simulink library "lib_fuel_converter3"  (Simulink 10.1)
settings: Solver=VariableStepAuto  StartTime=0.0  StopTime=10.0  RelTol=1e-3
undefined symbols (not defined in the file or in its folder): air_cp, amb_tmp, cyc_mph, ex_gas_cp, fc_acc_mass, fc_base_mass, fc_c2i_th_cond, fc_c_init_tmp, fc_cl2h_eff, fc_CO2_to_FUELgps, fc_cold, fc_cold_tmp, fc_cp, fc_ct_trq, fc_emisv, fc_ext_sarea, fc_fuel_den, fc_fuel_lhv, fc_h2x_th_cond, fc_h_air_flow, fc_h_cp, fc_h_init_tmp, fc_hood_emisv, fc_hood_sarea, fc_i2x_th_cond, fc_i_init_tmp, fc_inertia, fc_map_spd, fc_map_trq, fc_max_trq, fc_pwr_scale, fc_spd_scale, fc_trq_scale, fc_tstat, fc_x_init_tmp, fd_ratio, gb_num_init, gb_ratio, pow, vc_idle_bool, vc_idle_spd, vc_key_on, veh_glider_mass, wh_radius
undefined symbols (not defined in the file): fc_co_map, fc_co_map_c2h, fc_exflow_map, fc_extmp_map, fc_fuel_map, fc_fuel_map_c2h, fc_hc_map, fc_hc_map_c2h, fc_nn_model_name, fc_nox_map, fc_nox_map_c2h, fc_o2_map, fc_pm_map, fc_pm_map_c2h, generalName, logFlag
libraries: $bdroot x4, lib_etc x4, lib_fuel_converter x2, lib_fuel_converter2 x1
(part 4 of 8)

== system lib_fuel_converter3/configurable subsystems/fuel use and EO emis/fc temp correct/fc temp correct Variable Correction Factors (Map Based) ==
  Coolant T (C) : Inport
  HOT fuel use (g/s) : Inport  Port=2
  HOT emis (g/s) : Inport  Port=3
  T (Nm) : Inport  Port=4
  w (rad/s) : Inport  Port=5
  Enable : EnablePort  StatesWhenEnabling=reset
  (Thot-Temp) -------------------- (Thot-Tcold) : Fcn  Expr=(fc_tstat-u)/(fc_tstat-fc_cold_tmp)
  CO factor cold-to-hot : Subsystem  mask(2-D Table Lookup){xindex=fc_map_spd*fc_spd_scale, yindex=fc_map_trq*fc_trq_scale, table=fc_co_map_c2h}
      mask prompts: xindex "X Index"; yindex "Y Index"
      mask help:
      | Two Dimensional Table Lookup
      | The first input corresponds to X Index and the second input corresponds to the Y Index
      mask init:
      | sftab2chk(xindex,yindex,table);
      mask Help: This block returns a linearly interpolated intersection from the table using the X index (which corresponds to the rows of the table) and the Y index (which corresponds to the columns of the table).  Extrapolation is used.
      mask Display: plot(-10,-10,110,110,[90,50,10],[90,40,30],[90,50,10],[50,26,20],[90,50,10],[22,13,10])
  HC factor cold-to-hot : Subsystem  mask(2-D Table Lookup){xindex=fc_map_spd*fc_spd_scale, yindex=fc_map_trq*fc_trq_scale, table=fc_hc_map_c2h}
      mask prompts: xindex "X Index"; yindex "Y Index"
      mask help:
      | Two Dimensional Table Lookup
      | The first input corresponds to X Index and the second input corresponds to the Y Index
      mask init:
      | sftab2chk(xindex,yindex,table);
      mask Help: This block returns a linearly interpolated intersection from the table using the X index (which corresponds to the rows of the table) and the Y index (which corresponds to the columns of the table).  Extrapolation is used.
      mask Display: plot(-10,-10,110,110,[90,50,10],[90,40,30],[90,50,10],[50,26,20],[90,50,10],[22,13,10])
  Mux{1..5} (5 alike) : Mux  Inputs=2
  Mux6 : Mux
  NOx factor cold-to-hot : Subsystem  mask(2-D Table Lookup){xindex=fc_map_spd*fc_spd_scale, yindex=fc_map_trq*fc_trq_scale, table=fc_nox_map_c2h}
      mask prompts: xindex "X Index"; yindex "Y Index"
      mask help:
      | Two Dimensional Table Lookup
      | The first input corresponds to X Index and the second input corresponds to the Y Index
      mask init:
      | sftab2chk(xindex,yindex,table);
      mask Help: This block returns a linearly interpolated intersection from the table using the X index (which corresponds to the rows of the table) and the Y index (which corresponds to the columns of the table).  Extrapolation is used.
      mask Display: plot(-10,-10,110,110,[90,50,10],[90,40,30],[90,50,10],[50,26,20],[90,50,10],[22,13,10])
  PM factor cold-to-hot : Subsystem  mask(2-D Table Lookup){xindex=fc_map_spd*fc_spd_scale, yindex=fc_map_trq*fc_trq_scale, table=fc_pm_map_c2h}
      mask prompts: xindex "X Index"; yindex "Y Index"
      mask help:
      | Two Dimensional Table Lookup
      | The first input corresponds to X Index and the second input corresponds to the Y Index
      mask init:
      | sftab2chk(xindex,yindex,table);
      mask Help: This block returns a linearly interpolated intersection from the table using the X index (which corresponds to the rows of the table) and the Y index (which corresponds to the columns of the table).  Extrapolation is used.
      mask Display: plot(-10,-10,110,110,[90,50,10],[90,40,30],[90,50,10],[50,26,20],[90,50,10],[22,13,10])
  Product : Product  SaturateOnIntegerOverflow=on
  Product1 : Product  SaturateOnIntegerOverflow=on
  Saturation1 : Saturate  UpperLimit=max(fc_map_trq*fc_trq_scale)  LowerLimit=min(fc_map_trq*fc_trq_scale)
  Saturation2 : Saturate  UpperLimit=max(fc_map_spd*fc_spd_scale)  LowerLimit=min(fc_map_spd*fc_spd_scale)
  cold/hot =1+(factor-1) *Temp_ratio{,1..4} (5 alike) : Fcn  Expr=1+(u[2]-1)*u[1]
  fuel factor cold-to-hot : Subsystem  mask(2-D Table Lookup){xindex=fc_map_spd*fc_spd_scale, yindex=fc_map_trq*fc_trq_scale, table=fc_fuel_map_c2h}
      mask prompts: xindex "X Index"; yindex "Y Index"
      mask help:
      | Two Dimensional Table Lookup
      | The first input corresponds to X Index and the second input corresponds to the Y Index
      mask init:
      | sftab2chk(xindex,yindex,table);
      mask Help: This block returns a linearly interpolated intersection from the table using the X index (which corresponds to the rows of the table) and the Y index (which corresponds to the columns of the table).  Extrapolation is used.
      mask Display: plot(-10,-10,110,110,[90,50,10],[90,40,30],[90,50,10],[50,26,20],[90,50,10],[22,13,10])
  limit to data limits : Saturate  UpperLimit=1  LowerLimit=0
  fuel use (g/s) : Outport  OutputWhenDisabled=reset  InitialOutput=0
  EO emis (g/s) : Outport  Port=2  OutputWhenDisabled=reset  InitialOutput=0
  wires:
  cold/hot =1+(factor-1) *Temp_ratio4/1 -> Mux6/4
  cold/hot =1+(factor-1) *Temp_ratio3/1 -> Mux6/3
  cold/hot =1+(factor-1) *Temp_ratio2/1 -> Mux6/2
  cold/hot =1+(factor-1) *Temp_ratio1/1 -> Mux6/1
  cold/hot =1+(factor-1) *Temp_ratio/1 -> Product1/2
  limit to data limits/1 -> Mux5/1, Mux4/1, Mux3/1, Mux2/1, Mux1/1
  (Thot-Temp) -------------------- (Thot-Tcold)/1 -> limit to data limits/1
  Mux6/1 -> Product/1
  w (rad/s)/1 -> Saturation2/1
  T (Nm)/1 -> Saturation1/1
  HOT emis (g/s)/1 -> Product/2
  Product/1 -> EO emis (g/s)/1
  Product1/1 -> fuel use (g/s)/1
  Mux5/1 -> cold/hot =1+(factor-1) *Temp_ratio4/1
  Mux4/1 -> cold/hot =1+(factor-1) *Temp_ratio3/1
  Mux3/1 -> cold/hot =1+(factor-1) *Temp_ratio2/1
  Mux2/1 -> cold/hot =1+(factor-1) *Temp_ratio1/1
  PM factor cold-to-hot/1(table out) -> Mux5/2
  NOx factor cold-to-hot/1(table out) -> Mux4/2
  CO factor cold-to-hot/1(table out) -> Mux3/2
  HC factor cold-to-hot/1(table out) -> Mux2/2
  Mux1/1 -> cold/hot =1+(factor-1) *Temp_ratio/1
  fuel factor cold-to-hot/1(table out) -> Mux1/2
  Coolant T (C)/1 -> (Thot-Temp) -------------------- (Thot-Tcold)/1
  Saturation1/1 -> PM factor cold-to-hot/2(y0), NOx factor cold-to-hot/2(y0), CO factor cold-to-hot/2(y0), HC factor cold-to-hot/2(y0), fuel factor cold-to-hot/2(y0)
  Saturation2/1 -> PM factor cold-to-hot/1(x0), NOx factor cold-to-hot/1(x0), CO factor cold-to-hot/1(x0), HC factor cold-to-hot/1(x0), fuel factor cold-to-hot/1(x0)
  HOT fuel use (g/s)/1 -> Product1/1

== system lib_fuel_converter3/configurable subsystems/fuel use and EO emis Neural Network Model/HOT engine maps/Block NOTES ==
  note: This block determines the fully hot fuel use, engine-out emissions output rates, exhaust gas mass flow rate,
      | and engine-out exhaust gas temperature as a function of engine output torque and speed.
      | The engine maps (except for exhaust gas temperature) can be scaled using variables fc_spd_scale and
      |  fc_trq_scale; it is recommended that scaling values outside the range of 0.85 to 1.15 be used CAREFULLY.

== system lib_fuel_converter3/configurable subsystems/fuel use and EO emis Neural Network Model/HOT engine maps/CO (g/s) ==
  x0 : Inport
  y0 : Inport  Port=2
  Mux : Mux  Inputs=2
  S-function : S-Function  FunctionName=sftable2  Parameters=xindex, yindex, table  SFunctionDeploymentMode=off  EnableBusSupport=off
  table out : Outport  InitialOutput=0
  wires:
  y0/1 -> Mux/2
  S-function/1 -> table out/1
  x0/1 -> Mux/1
  Mux/1 -> S-function/1

== system lib_fuel_converter3/configurable subsystems/fuel use and EO emis Neural Network Model/HOT engine maps/HC (g/s) ==
  x0 : Inport
  y0 : Inport  Port=2
  Mux : Mux  Inputs=2
  S-function : S-Function  FunctionName=sftable2  Parameters=xindex, yindex, table  SFunctionDeploymentMode=off  EnableBusSupport=off
  table out : Outport  InitialOutput=0
  wires:
  y0/1 -> Mux/2
  S-function/1 -> table out/1
  x0/1 -> Mux/1
  Mux/1 -> S-function/1

== system lib_fuel_converter3/configurable subsystems/fuel use and EO emis Neural Network Model/HOT engine maps/MF,ex (g/s) ==
  x0 : Inport
  y0 : Inport  Port=2
  Mux : Mux  Inputs=2
  S-function : S-Function  FunctionName=sftable2  Parameters=xindex, yindex, table  SFunctionDeploymentMode=off  EnableBusSupport=off
  table out : Outport  InitialOutput=0
  wires:
  y0/1 -> Mux/2
  S-function/1 -> table out/1
  x0/1 -> Mux/1
  Mux/1 -> S-function/1

== system lib_fuel_converter3/configurable subsystems/fuel use and EO emis Neural Network Model/HOT engine maps/NOx (g/s) ==
  x0 : Inport
  y0 : Inport  Port=2
  Mux : Mux  Inputs=2
  S-function : S-Function  FunctionName=sftable2  Parameters=xindex, yindex, table  SFunctionDeploymentMode=off  EnableBusSupport=off
  table out : Outport  InitialOutput=0
  wires:
  y0/1 -> Mux/2
  S-function/1 -> table out/1
  x0/1 -> Mux/1
  Mux/1 -> S-function/1

== system lib_fuel_converter3/configurable subsystems/fuel use and EO emis Neural Network Model/HOT engine maps/O2 (g/s) ==
  x0 : Inport
  y0 : Inport  Port=2
  Mux : Mux  Inputs=2
  S-function : S-Function  FunctionName=sftable2  Parameters=xindex, yindex, table  SFunctionDeploymentMode=off  EnableBusSupport=off
  table out : Outport  InitialOutput=0
  wires:
  Mux/1 -> S-function/1
  x0/1 -> Mux/1
  S-function/1 -> table out/1
  y0/1 -> Mux/2

== system lib_fuel_converter3/configurable subsystems/fuel use and EO emis Neural Network Model/HOT engine maps/PM (g/s) ==
  x0 : Inport
  y0 : Inport  Port=2
  Mux : Mux  Inputs=2
  S-function : S-Function  FunctionName=sftable2  Parameters=xindex, yindex, table  SFunctionDeploymentMode=off  EnableBusSupport=off
  table out : Outport  InitialOutput=0
  wires:
  y0/1 -> Mux/2
  S-function/1 -> table out/1
  x0/1 -> Mux/1
  Mux/1 -> S-function/1

== system lib_fuel_converter3/configurable subsystems/fuel use and EO emis Neural Network Model/HOT engine maps/Tex,eo (C) ==
  x0 : Inport
  y0 : Inport  Port=2
  Mux : Mux  Inputs=2
  S-function : S-Function  FunctionName=sftable2  Parameters=xindex, yindex, table  SFunctionDeploymentMode=off  EnableBusSupport=off
  table out : Outport  InitialOutput=0
  wires:
  y0/1 -> Mux/2
  S-function/1 -> table out/1
  x0/1 -> Mux/1
  Mux/1 -> S-function/1

== system lib_fuel_converter3/configurable subsystems/fuel use and EO emis Neural Network Model/HOT engine maps/fuel (g/s) ==
  x0 : Inport
  y0 : Inport  Port=2
  Mux : Mux  Inputs=2
  S-function : S-Function  FunctionName=sftable2  Parameters=xindex, yindex, table  SFunctionDeploymentMode=off  EnableBusSupport=off
  table out : Outport  InitialOutput=0
  wires:
  y0/1 -> Mux/2
  S-function/1 -> table out/1
  x0/1 -> Mux/1
  Mux/1 -> S-function/1

== system lib_fuel_converter3/configurable subsystems/fuel use and EO emis Neural Network Model/fc temp/Block NOTES ==
  note: This block models the thermal behavior internal combustion engine (ICE).
      | Emphasis is on the coolant since this temperature is used to correct engine
      | fuel use.

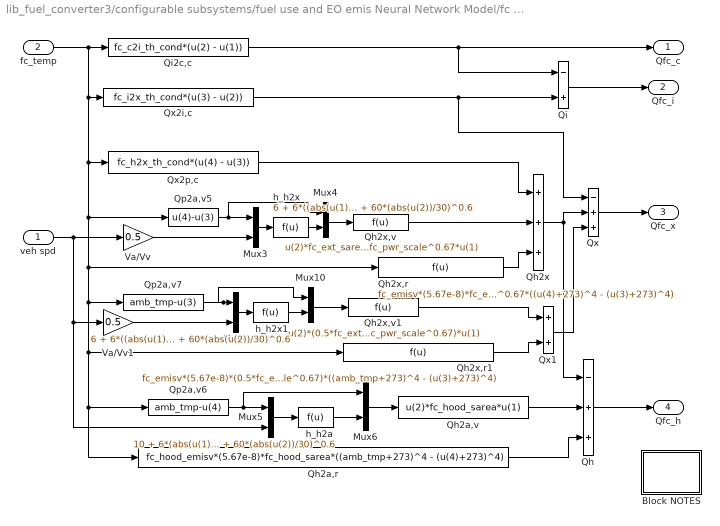
== system lib_fuel_converter3/configurable subsystems/fuel use and EO emis Neural Network Model/fc temp/fc mass heat flow ==
  veh spd : Inport
  fc_temp : Inport  Port=2
  Block NOTES : Subsystem
      mask Display: disp('Block\nNOTES')
  Mux{3..6,9..10} (6 alike) : Mux  Inputs=2
  Qh : Sum  Inputs=-++  SaturateOnIntegerOverflow=on
  Qh2a,r : Fcn  Expr=fc_hood_emisv*(5.67e-8)*fc_hood_sarea*((amb_tmp+273)^4 - (u(4)+273)^4)
  Qh2a,v : Fcn  Expr=u(2)*fc_hood_sarea*u(1)
  Qh2x : Sum  Inputs=+++  SaturateOnIntegerOverflow=on
  Qh2x,r : Fcn  Expr=fc_emisv*(5.67e-8)*fc_ext_sarea*fc_pwr_scale^0.67*((u(4)+273)^4 - (u(3)+273)^4)
  Qh2x,r1 : Fcn  Expr=fc_emisv*(5.67e-8)*(0.5*fc_ext_sarea*fc_pwr_scale^0.67)*((amb_tmp+273)^4 - (u(3)+273)^4)
  Qh2x,v : Fcn  Expr=u(2)*fc_ext_sarea*fc_pwr_scale^0.67*u(1)
  Qh2x,v1 : Fcn  Expr=u(2)*(0.5*fc_ext_sarea*fc_pwr_scale^0.67)*u(1)
  Qi : Sum  Inputs=-+  SaturateOnIntegerOverflow=on
  Qi2c,c : Fcn  Expr=fc_c2i_th_cond*(u(2) - u(1))
  Qp2a,v5 : Fcn  Expr=u(4)-u(3)
  Qp2a,v6 : Fcn  Expr=amb_tmp-u(4)
  Qp2a,v7 : Fcn  Expr=amb_tmp-u(3)
  Qx : Sum  Inputs=-++  SaturateOnIntegerOverflow=on
  Qx1 : Sum  SaturateOnIntegerOverflow=on
  Qx2i,c : Fcn  Expr=fc_i2x_th_cond*(u(3) - u(2))
  Qx2p,c : Fcn  Expr=fc_h2x_th_cond*(u(4) - u(3))
  Va/Vv : Gain  Gain=0.5  SaturateOnIntegerOverflow=on
  Va/Vv1 : Gain  Gain=0.5  SaturateOnIntegerOverflow=on
  h_h2a : Fcn  Expr=10 + 6*(abs(u(1))/1000)^0.3 + 60*(abs(u(2))/30)^0.6
  h_h2x : Fcn  Expr=6 + 6*((abs(u(1))/1000))^0.3 + 60*(abs(u(2))/30)^0.6
  h_h2x1 : Fcn  Expr=6 + 6*((abs(u(1))/1000))^0.3 + 60*(abs(u(2))/30)^0.6
  Qfc_c : Outport
  Qfc_i : Outport  Port=2
  Qfc_x : Outport  Port=3
  Qfc_h : Outport  Port=4
  wires:
  Mux10/1 -> Qh2x,v1/1
  Mux9/1 -> h_h2x1/1
  Qp2a,v7/1 -> Mux9/1, Mux10/1
  h_h2x1/1 -> Mux10/2
  Va/Vv1/1 -> Mux9/2
  Mux4/1 -> Qh2x,v/1
  Mux3/1 -> h_h2x/1
  Qp2a,v5/1 -> Mux3/1, Mux4/1
  h_h2x/1 -> Mux4/2
  veh spd/1 -> Va/Vv/1, Mux5/2, Va/Vv1/1
  Va/Vv/1 -> Mux3/2
  Qi2c,c/1 -> Qfc_c/1, Qi/1
  fc_temp/1 -> Qx2p,c/1, Qh2x,r/1, Qp2a,v7/1, Qp2a,v6/1, Qh2a,r/1, Qh2x,r1/1, Qp2a,v5/1, Qx2i,c/1, Qi2c,c/1
  Qx2i,c/1 -> Qi/2, Qx/1
  Qi/1 -> Qfc_i/1
  Qx/1 -> Qfc_x/1
  Qh2x/1 -> Qx/2, Qh/1
  Qh/1 -> Qfc_h/1
  Mux6/1 -> Qh2a,v/1
  Mux5/1 -> h_h2a/1
  Qp2a,v6/1 -> Mux5/1, Mux6/1
  h_h2a/1 -> Mux6/2
  Qx1/1 -> Qx/3
  Qh2x,v/1 -> Qh2x/2
  Qx2p,c/1 -> Qh2x/1
  Qh2x,r1/1 -> Qx1/2
  Qh2x,v1/1 -> Qx1/1
  Qh2a,r/1 -> Qh/3
  Qh2a,v/1 -> Qh/2
  Qh2x,r/1 -> Qh2x/3

== system lib_fuel_converter3/configurable subsystems/fuel use and EO emis Neural Network Model/fc temp/old fc coolant  temp. (C) ==
  fc on? : Inport
  veh spd : Inport  Port=2
  Block NOTES : Subsystem
      mask Display: disp('Block\nNOTES')
  Mux : Mux
  TEC : Integrator  InitialCondition=fc_i_init_tmp
  compute engine dT/dt : Fcn  Expr=1.1*u[1]*(-u[2]/218)*(95-u[4])+(1-u[1])*u[3]*(u[4]-amb_tmp)
  gamma (takes v as input) : Fcn  Expr=(-8.22e-5*u+8.09e-6*4-1.45e-4)*.45
  log(1-40/75) : Constant  Value=-0.7621
  fc coolant  temp (C) : Outport  InitialOutput=0
  wires:
  compute engine dT/dt/1 -> TEC/1
  gamma (takes v as input)/1 -> Mux/3
  log(1-40/75)/1 -> Mux/2
  Mux/1 -> compute engine dT/dt/1
  fc on?/1 -> Mux/1
  veh spd/1 -> gamma (takes v as input)/1
  TEC/1 -> fc coolant  temp (C)/1, Mux/4

== system lib_fuel_converter3/configurable subsystems/fuel use and EO emis Neural Network Model/fc temp correct/fc temp correct Constant Correction Factors (Equation Based) ==
  Coolant T (C) : Inport
  HOT fuel use (g/s) : Inport  Port=2
  HOT emis (g/s) : Inport  Port=3
  Enable : EnablePort  StatesWhenEnabling=reset
  Block NOTES : Subsystem
      mask Display: disp('Block\nNOTES')
  CO cold/hot : Fcn  Expr=2.13*pow(u,4.26)+1
  HC cold/hot : Fcn  Expr=8.05*pow(u,9.46)+1
  Mux : Mux
  NOx cold/hot : Fcn  Expr=0.51*pow(u,1.37)+1
  PM cold/hot : Fcn  Expr=5.14*pow(u,17.04)+1
  Product : Product  SaturateOnIntegerOverflow=on
  Product1 : Product  SaturateOnIntegerOverflow=on
  Saturation : Saturate  UpperLimit=1  LowerLimit=0
  fuel cold/hot : Fcn  Expr=0.1*pow(u,0.65)+1
  lambda : Fcn  Expr=(fc_tstat-u)/(fc_tstat-20)
  fuel use (g/s) : Outport  OutputWhenDisabled=reset  InitialOutput=0
  EO emis (g/s) : Outport  Port=2  OutputWhenDisabled=reset  InitialOutput=0
  wires:
  PM cold/hot/1 -> Mux/4
  NOx cold/hot/1 -> Mux/3
  HC cold/hot/1 -> Mux/1
  Saturation/1 -> CO cold/hot/1, HC cold/hot/1, fuel cold/hot/1, NOx cold/hot/1, PM cold/hot/1
  lambda/1 -> Saturation/1
  Mux/1 -> Product/1
  fuel cold/hot/1 -> Product1/2
  Product/1 -> EO emis (g/s)/1
  CO cold/hot/1 -> Mux/2
  Product1/1 -> fuel use (g/s)/1
  HOT fuel use (g/s)/1 -> Product1/1
  Coolant T (C)/1 -> lambda/1
  HOT emis (g/s)/1 -> Product/2

== system lib_fuel_converter3/configurable subsystems/fuel use and EO emis Neural Network Model/fc temp correct/fc temp correct Variable Correction Factors (Map Based) ==
  Coolant T (C) : Inport
  HOT fuel use (g/s) : Inport  Port=2
  HOT emis (g/s) : Inport  Port=3
  T (Nm) : Inport  Port=4
  w (rad/s) : Inport  Port=5
  Enable : EnablePort  StatesWhenEnabling=reset
  (Thot-Temp) -------------------- (Thot-Tcold) : Fcn  Expr=(fc_tstat-u)/(fc_tstat-fc_cold_tmp)
  CO factor cold-to-hot : Subsystem  mask(2-D Table Lookup){xindex=fc_map_spd*fc_spd_scale, yindex=fc_map_trq*fc_trq_scale, table=fc_co_map_c2h}
      mask prompts: xindex "X Index"; yindex "Y Index"
      mask help:
      | Two Dimensional Table Lookup
      | The first input corresponds to X Index and the second input corresponds to the Y Index
      mask init:
      | sftab2chk(xindex,yindex,table);
      mask Help: This block returns a linearly interpolated intersection from the table using the X index (which corresponds to the rows of the table) and the Y index (which corresponds to the columns of the table).  Extrapolation is used.
      mask Display: plot(-10,-10,110,110,[90,50,10],[90,40,30],[90,50,10],[50,26,20],[90,50,10],[22,13,10])
  HC factor cold-to-hot : Subsystem  mask(2-D Table Lookup){xindex=fc_map_spd*fc_spd_scale, yindex=fc_map_trq*fc_trq_scale, table=fc_hc_map_c2h}
      mask prompts: xindex "X Index"; yindex "Y Index"
      mask help:
      | Two Dimensional Table Lookup
      | The first input corresponds to X Index and the second input corresponds to the Y Index
      mask init:
      | sftab2chk(xindex,yindex,table);
      mask Help: This block returns a linearly interpolated intersection from the table using the X index (which corresponds to the rows of the table) and the Y index (which corresponds to the columns of the table).  Extrapolation is used.
      mask Display: plot(-10,-10,110,110,[90,50,10],[90,40,30],[90,50,10],[50,26,20],[90,50,10],[22,13,10])
  Mux{1..5} (5 alike) : Mux  Inputs=2
  Mux6 : Mux
  NOx factor cold-to-hot : Subsystem  mask(2-D Table Lookup){xindex=fc_map_spd*fc_spd_scale, yindex=fc_map_trq*fc_trq_scale, table=fc_nox_map_c2h}
      mask prompts: xindex "X Index"; yindex "Y Index"
      mask help:
      | Two Dimensional Table Lookup
      | The first input corresponds to X Index and the second input corresponds to the Y Index
      mask init:
      | sftab2chk(xindex,yindex,table);
      mask Help: This block returns a linearly interpolated intersection from the table using the X index (which corresponds to the rows of the table) and the Y index (which corresponds to the columns of the table).  Extrapolation is used.
      mask Display: plot(-10,-10,110,110,[90,50,10],[90,40,30],[90,50,10],[50,26,20],[90,50,10],[22,13,10])
  PM factor cold-to-hot : Subsystem  mask(2-D Table Lookup){xindex=fc_map_spd*fc_spd_scale, yindex=fc_map_trq*fc_trq_scale, table=fc_pm_map_c2h}
      mask prompts: xindex "X Index"; yindex "Y Index"
      mask help:
      | Two Dimensional Table Lookup
      | The first input corresponds to X Index and the second input corresponds to the Y Index
      mask init:
      | sftab2chk(xindex,yindex,table);
      mask Help: This block returns a linearly interpolated intersection from the table using the X index (which corresponds to the rows of the table) and the Y index (which corresponds to the columns of the table).  Extrapolation is used.
      mask Display: plot(-10,-10,110,110,[90,50,10],[90,40,30],[90,50,10],[50,26,20],[90,50,10],[22,13,10])
  Product : Product  SaturateOnIntegerOverflow=on
  Product1 : Product  SaturateOnIntegerOverflow=on
  Saturation1 : Saturate  UpperLimit=max(fc_map_trq*fc_trq_scale)  LowerLimit=min(fc_map_trq*fc_trq_scale)
  Saturation2 : Saturate  UpperLimit=max(fc_map_spd*fc_spd_scale)  LowerLimit=min(fc_map_spd*fc_spd_scale)
  cold/hot =1+(factor-1) *Temp_ratio{,1..4} (5 alike) : Fcn  Expr=1+(u[2]-1)*u[1]
  fuel factor cold-to-hot : Subsystem  mask(2-D Table Lookup){xindex=fc_map_spd*fc_spd_scale, yindex=fc_map_trq*fc_trq_scale, table=fc_fuel_map_c2h}
      mask prompts: xindex "X Index"; yindex "Y Index"
      mask help:
      | Two Dimensional Table Lookup
      | The first input corresponds to X Index and the second input corresponds to the Y Index
      mask init:
      | sftab2chk(xindex,yindex,table);
      mask Help: This block returns a linearly interpolated intersection from the table using the X index (which corresponds to the rows of the table) and the Y index (which corresponds to the columns of the table).  Extrapolation is used.
      mask Display: plot(-10,-10,110,110,[90,50,10],[90,40,30],[90,50,10],[50,26,20],[90,50,10],[22,13,10])
  limit to data limits : Saturate  UpperLimit=1  LowerLimit=0
  fuel use (g/s) : Outport  OutputWhenDisabled=reset  InitialOutput=0
  EO emis (g/s) : Outport  Port=2  OutputWhenDisabled=reset  InitialOutput=0
  wires:
  cold/hot =1+(factor-1) *Temp_ratio4/1 -> Mux6/4
  cold/hot =1+(factor-1) *Temp_ratio3/1 -> Mux6/3
  cold/hot =1+(factor-1) *Temp_ratio2/1 -> Mux6/2
  cold/hot =1+(factor-1) *Temp_ratio1/1 -> Mux6/1
  cold/hot =1+(factor-1) *Temp_ratio/1 -> Product1/2
  limit to data limits/1 -> Mux5/1, Mux4/1, Mux3/1, Mux2/1, Mux1/1
  (Thot-Temp) -------------------- (Thot-Tcold)/1 -> limit to data limits/1
  Mux6/1 -> Product/1
  w (rad/s)/1 -> Saturation2/1
  T (Nm)/1 -> Saturation1/1
  HOT emis (g/s)/1 -> Product/2
  Product/1 -> EO emis (g/s)/1
  Product1/1 -> fuel use (g/s)/1
  Mux5/1 -> cold/hot =1+(factor-1) *Temp_ratio4/1
  Mux4/1 -> cold/hot =1+(factor-1) *Temp_ratio3/1
  Mux3/1 -> cold/hot =1+(factor-1) *Temp_ratio2/1
  Mux2/1 -> cold/hot =1+(factor-1) *Temp_ratio1/1
  PM factor cold-to-hot/1(table out) -> Mux5/2
  NOx factor cold-to-hot/1(table out) -> Mux4/2
  CO factor cold-to-hot/1(table out) -> Mux3/2
  HC factor cold-to-hot/1(table out) -> Mux2/2
  Mux1/1 -> cold/hot =1+(factor-1) *Temp_ratio/1
  fuel factor cold-to-hot/1(table out) -> Mux1/2
  Coolant T (C)/1 -> (Thot-Temp) -------------------- (Thot-Tcold)/1
  Saturation1/1 -> PM factor cold-to-hot/2(y0), NOx factor cold-to-hot/2(y0), CO factor cold-to-hot/2(y0), HC factor cold-to-hot/2(y0), fuel factor cold-to-hot/2(y0)
  Saturation2/1 -> PM factor cold-to-hot/1(x0), NOx factor cold-to-hot/1(x0), CO factor cold-to-hot/1(x0), HC factor cold-to-hot/1(x0), fuel factor cold-to-hot/1(x0)
  HOT fuel use (g/s)/1 -> Product1/1

== system lib_fuel_converter3/fuel converter  <fc> for series/Model & Interface/model/Block NOTES ==
  note: This block models the internal combustion engine, and includes inertia effects,
      | performance limits, accessory loads, and temperature transient effects on fuel
      | use, engine-out emissions, and catalyst efficiency.  There are 'leads' to the
      | engine controller here, which controller determines whether the engine is on.

== system lib_fuel_converter3/fuel converter  <fc> for series/Model & Interface/model/enhancedToWorkspace ==
  In1 : Inport
  To Workspace : ToWorkspace  VariableName=fc_spd_out_r  SampleTime=-1
  wires:
  In1/1 -> To Workspace/1

== system lib_fuel_converter3/fuel converter  <fc> for series/Model & Interface/model/enhancedToWorkspace1 ==
  In1 : Inport
  To Workspace : ToWorkspace  VariableName=fc_trq_out_r  SampleTime=-1
  wires:
  In1/1 -> To Workspace/1

== system lib_fuel_converter3/fuel converter  <fc> for series/Model & Interface/model/enhancedToWorkspace2 ==
  In1 : Inport
  To Workspace : ToWorkspace  VariableName=fc_spd_est  SampleTime=-1
  wires:
  In1/1 -> To Workspace/1

== system lib_fuel_converter3/fuel converter  <fc> for series/Model & Interface/model/enhancedToWorkspace3 ==
  In1 : Inport
  To Workspace : ToWorkspace  VariableName=fc_brake_trq  SampleTime=-1
  wires:
  In1/1 -> To Workspace/1

== system lib_fuel_converter3/fuel converter  <fc> for series/Model & Interface/model/fuel use and EO emis Configurable Subsystem ==
  T (Nm) : Inport
  w (rad/s) : Inport  Port=2
  fuel use and EO emis : $bdroot/configurable subsystems/fuel use and EO emis
      settings: RTWFcnNameOpts=Auto  RTWFileNameOpts=Auto
  cumulative fuel  use (gal) : Outport
  "FC ON?, EOem, MFex, Tex, O2ex" : Outport  Port=2
  Vv,Tfc : Outport  Port=3
  wires:
  T (Nm)/1 -> fuel use and EO emis/1
  w (rad/s)/1 -> fuel use and EO emis/2
  fuel use and EO emis/1 -> cumulative fuel  use (gal)/1
  fuel use and EO emis/2 -> "FC ON?, EOem, MFex, Tex, O2ex"/1
  fuel use and EO emis/3 -> Vv,Tfc/1

== system lib_fuel_converter3/fuel converter  <fc> for series/Model & Interface/model/help ==

== system lib_fuel_converter3/fuel converter  <fc> for series/Model & Interface/model/providing trq (+ive or -ive) ==
  req'd trq (Nm) : Inport
  req'd spd (rad/s) : Inport  Port=2
  prev engine spd (rad/s) : Inport  Port=3
  Mux3 : Mux  Inputs=3
  Sum1 : Sum  Inputs=+-  SaturateOnIntegerOverflow=on
  Sum2 : Sum  SaturateOnIntegerOverflow=on
  effect of inertia (Nm) : Subsystem
  enforce engine limits : Subsystem
  map trq (Nm) spd (rad/s) trq to drivetrain (Nm) : Outport  InitialOutput=0
  wires:
  req'd spd (rad/s)/1 -> enforce engine limits/2(req'd engine spd (rad/s))
  Sum1/1 -> Mux3/3
  Mux3/1 -> map trq (Nm) spd (rad/s) trq to drivetrain (Nm)/1
  prev engine spd (rad/s)/1 -> effect of inertia (Nm)/2(prev spd)
  enforce engine limits/1(limited engine brake trq (Nm)) -> Mux3/1, Sum1/1
  enforce engine limits/2(limited engine spd (rad/s)) -> effect of inertia (Nm)/1(req'd spd (rad/s)), Mux3/2
  req'd trq (Nm)/1 -> Sum2/1
  effect of inertia (Nm)/1((Nm)) -> Sum1/2, Sum2/2
  Sum2/1 -> enforce engine limits/1(req'd engine trq (Nm))

== system lib_fuel_converter3/fuel converter  <fc> for series/Model & Interface/model/spinning up or spinning down ==
  spd command (rad/s) : Inport
  engine disconnected from drivetrain : Inport  Port=2
  previous engine spd (rad/s) : Inport  Port=3
  Constant : Constant  Value=0
  Constant1 : Constant  Value=vc_idle_spd
  MinMax : MinMax  Inputs=2
  MinMax1 : MinMax  Function=max  Inputs=2
  Mux3 : Mux  Inputs=3
  Product : Product  SaturateOnIntegerOverflow=on
  Product2 : Product  SaturateOnIntegerOverflow=on
  Relational Operator : RelationalOperator  Operator=<=  RndMeth=Nearest  InputSameDT=on
  Sum : Sum  Inputs=|++  SaturateOnIntegerOverflow=on
  Sum1 : Sum  Inputs=|+-  SaturateOnIntegerOverflow=on
  Sum2 : Sum  SaturateOnIntegerOverflow=on
  Switch: map torque : Switch  Threshold=eps  SaturateOnIntegerOverflow=on  InputSameDT=on
  T_closed throttle : Subsystem
  T_max : Subsystem
  alpha : Gain  Gain=1/(fc_inertia+eps)  SaturateOnIntegerOverflow=on
  dt : Subsystem
  effect of inertia (Nm) : Subsystem
  just started spin-down/spin-up : Subsystem
  no-lag Reset Integrator : Subsystem  mask(No-lag Reset Integrator){initval=vc_idle_spd}
      mask prompts: initval "Initial Value"
      mask help: No-lag Reset Integrator
      mask Help: Integrates first input using Euler technique.\nAt the time step that input 2 <> zero,\noutput is reset to input 3.
      mask Display: disp('1/s\nw/ reset\nno lag')
  map trq (Nm) spd (rad/s) trq to drivetrain (Nm) : Outport  InitialOutput=0
  wires:
  [acc_mech_trq_est] -> Sum1/2
  Sum1/1 -> alpha/1
  [acc_mech_trq_est] -> Sum/2
  Sum/1 -> MinMax/2
  effect of inertia (Nm)/1((Nm)) -> Sum/1
  MinMax1/1 -> Mux3/2
  Product2/1 -> MinMax1/2
  [engine_on] -> Product2/2
  Constant1/1 -> Product2/1
  Constant/1 -> Mux3/3
  Mux3/1 -> map trq (Nm) spd (rad/s) trq to drivetrain (Nm)/1
  dt/1(out_1) -> Product/2
  Product/1 -> Sum2/1
  engine disconnected from drivetrain/1 -> just started spin-down/spin-up/1(state)
  Sum2/1 -> no-lag Reset Integrator/3(in_3)
  just started spin-down/spin-up/1(trigger) -> no-lag Reset Integrator/2(in_2)
  no-lag Reset Integrator/1(out_1) -> MinMax1/1
  spd command (rad/s)/1 -> effect of inertia (Nm)/1(req'd spd (rad/s)), Relational Operator/2
  previous engine spd (rad/s)/1 -> Sum2/2, Relational Operator/1, effect of inertia (Nm)/2(prev spd), T_max/1(w_APU), T_closed throttle/1(w_APU)
  alpha/1 -> no-lag Reset Integrator/1(in_1), Product/1
  Relational Operator/1 -> Switch: map torque/2
  Switch: map torque/1 -> Sum1/1, Mux3/1
  T_closed throttle/1(T_closed throttle) -> Switch: map torque/3
  MinMax/1 -> Switch: map torque/1
  T_max/1(T_max) -> MinMax/1

== system lib_fuel_converter3/fuel converter <fc>/IC Engine Model  &  Interface/ic engine model/Block NOTES ==
  note: This block models the internal combustion engine, and includes inertia effects,
      | performance limits, accessory loads, and temperature transient effects on fuel
      | use, engine-out emissions, and catalyst efficiency.  There are 'leads' to the
      | engine controller here, which controller determines whether the engine is on.

== system lib_fuel_converter3/fuel converter <fc>/IC Engine Model  &  Interface/ic engine model/Speed Limits ==
  Speed Requested : Inport
  Constant : Constant  Value=0
  Speed Limits : Saturate  UpperLimit=max(fc_map_spd)*fc_spd_scale  LowerLimit=vc_idle_spd*vc_idle_bool
  "if engine is not on, speed is zero" : Switch  Threshold=0.5  SaturateOnIntegerOverflow=on  InputSameDT=on
  Limited Speed Request : Outport
  wires:
  Speed Requested/1 -> Speed Limits/1
  Speed Limits/1 -> "if engine is not on, speed is zero"/1
  "if engine is not on, speed is zero"/1 -> Limited Speed Request/1
  [engine_on] -> "if engine is not on, speed is zero"/2
  Constant/1 -> "if engine is not on, speed is zero"/3

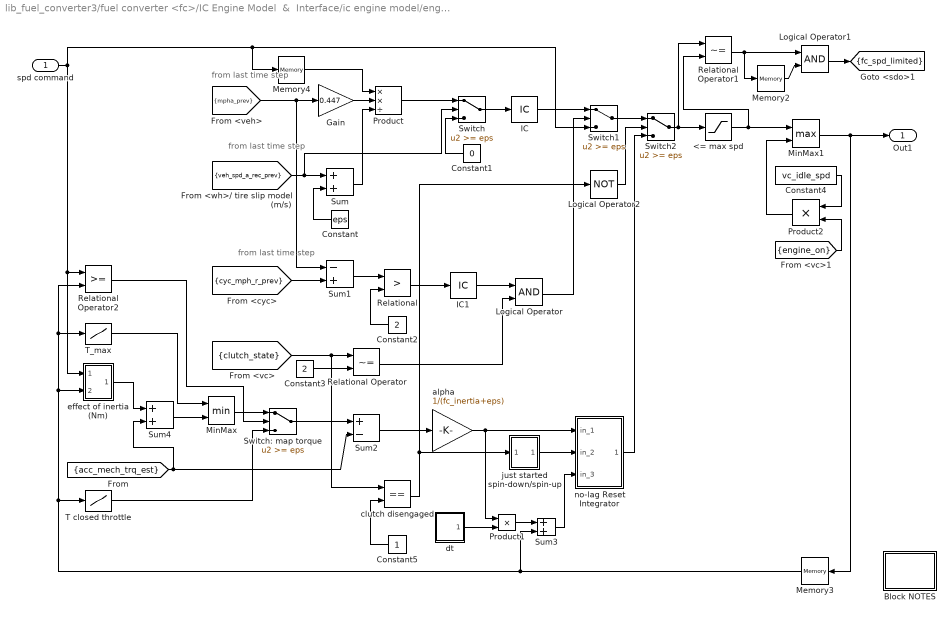
== system lib_fuel_converter3/fuel converter <fc>/IC Engine Model  &  Interface/ic engine model/engine speed estimator ==
  note: from last time step
  note: from last time step
  note: from last time step
  spd command : Inport
  <= max spd : Saturate  UpperLimit=max(fc_map_spd)*fc_spd_scale  LowerLimit=-inf
  Block NOTES : Subsystem
      mask Display: disp('Block\nNOTES')
  Constant : Constant  Value=eps
  Constant1 : Constant  Value=0
  Constant2 : Constant  Value=2
  Constant3 : Constant  Value=2
  Constant4 : Constant  Value=vc_idle_spd
  Constant5 : Constant
  Gain : Gain  Gain=0.447  SaturateOnIntegerOverflow=on
  IC : InitialCondition  Value=cyc_mph(1,2)*0.447/wh_radius*fd_ratio*gb_ratio(gb_num_init)
  IC1 : InitialCondition  Value=0
  Logical Operator : Logic
  Logical Operator1 : Logic
  Logical Operator2 : Logic  Operator=NOT  Inputs=1
  Memory2 : Memory
  Memory3 : Memory  InitialCondition=cyc_mph(1,2)*0.447/wh_radius*fd_ratio*max(gb_ratio)
  Memory4 : Memory
  MinMax : MinMax  Inputs=2
  MinMax1 : MinMax  Function=max  Inputs=2
  Product : Product  Inputs=**/  SaturateOnIntegerOverflow=on
  Product1 : Product  SaturateOnIntegerOverflow=on
  Product2 : Product  SaturateOnIntegerOverflow=on
  Relational : RelationalOperator  Operator=>  RndMeth=Nearest  InputSameDT=on
  Relational Operator : RelationalOperator  Operator=~=  RndMeth=Nearest  InputSameDT=on
  Relational Operator1 : RelationalOperator  Operator=~=  RndMeth=Nearest  InputSameDT=on
  Relational Operator2 : RelationalOperator  RndMeth=Nearest  InputSameDT=on
  Sum : Sum  SaturateOnIntegerOverflow=on
  Sum1 : Sum  Inputs=-+  SaturateOnIntegerOverflow=on
  Sum2 : Sum  Inputs=+-  SaturateOnIntegerOverflow=on
  Sum3 : Sum  SaturateOnIntegerOverflow=on
  Sum4 : Sum  SaturateOnIntegerOverflow=on
  Switch : Switch  Threshold=eps  SaturateOnIntegerOverflow=on  InputSameDT=on
  Switch1 : Switch  Threshold=eps  SaturateOnIntegerOverflow=on  InputSameDT=on
  Switch2 : Switch  Threshold=eps  SaturateOnIntegerOverflow=on  InputSameDT=on
  Switch: map torque : Switch  Threshold=eps  SaturateOnIntegerOverflow=on  InputSameDT=on
  T closed throttle : Lookup  InputValues=fc_map_spd*fc_spd_scale  Table=fc_ct_trq*fc_trq_scale  SaturateOnIntegerOverflow=on
  T_max : Lookup  InputValues=fc_map_spd*fc_spd_scale  Table=fc_max_trq*fc_trq_scale  SaturateOnIntegerOverflow=on
  alpha : Gain  Gain=1/(fc_inertia+eps)  SaturateOnIntegerOverflow=on
  clutch disengaged : RelationalOperator  Operator===  RndMeth=Nearest  InputSameDT=on
  dt : Subsystem
  effect of inertia (Nm) : Subsystem
  just started spin-down/spin-up : Subsystem
  no-lag Reset Integrator : Subsystem  mask(No-lag Reset Integrator){initval=vc_idle_spd}
      mask prompts: initval "Initial Value"
      mask help: No-lag Reset Integrator
      mask Help: Integrates first input using Euler technique.\nAt the time step that input 2 <> zero,\noutput is reset to input 3.
      mask Display: disp('1/s\nw/ reset\nno lag')
  Out1 : Outport
  tag scope: fc_spd_limited=scoped
  wires:
  IC1/1 -> Logical Operator/1
  Memory4/1 -> Product/1
  [acc_mech_trq_est] -> Sum2/2, Sum4/2
  Product/1 -> Switch/1
  [veh_spd_a_rec_prev] -> Sum/1, Switch/2
  Constant1/1 -> Switch/3
  IC/1 -> Switch1/1
  Constant/1 -> Sum/2
  [cyc_mph_r_prev] -> Sum1/2
  [mpha_prev] -> Gain/1, Sum1/1
  Constant2/1 -> Relational/2
  Sum1/1 -> Relational/1
  Relational/1 -> IC1/1
  Switch/1 -> IC/1
  Gain/1 -> Product/2
  Sum/1 -> Product/3
  Relational Operator/1 -> Logical Operator/2
  Constant3/1 -> Relational Operator/2
  Sum2/1 -> alpha/1
  dt/1(out_1) -> Product1/2
  Product1/1 -> Sum3/1
  alpha/1 -> Product1/1, no-lag Reset Integrator/1(in_1)
  Constant5/1 -> clutch disengaged/2
  Switch1/1 -> Switch2/1
  clutch disengaged/1 -> Logical Operator2/1, just started spin-down/spin-up/1(state)
  [clutch_state] -> Relational Operator/1, clutch disengaged/1
  Memory3/1 -> Sum3/2, Relational Operator2/2, T_max/1, effect of inertia (Nm)/2(prev spd), T closed throttle/1
  <= max spd/1 -> Relational Operator1/2, MinMax1/1
  [engine_on] -> Product2/2
  Constant4/1 -> Product2/1
  MinMax1/1 -> Out1/1, Memory3/1
  Product2/1 -> MinMax1/2
  Switch2/1 -> <= max spd/1, Relational Operator1/1
  Memory2/1 -> Logical Operator1/2
  Logical Operator1/1 -> [fc_spd_limited]
  Relational Operator1/1 -> Logical Operator1/1, Memory2/1
  Switch: map torque/1 -> Sum2/1
  Relational Operator2/1 -> Switch: map torque/2
  T closed throttle/1 -> Switch: map torque/3
  MinMax/1 -> Switch: map torque/1
  T_max/1 -> MinMax/1
  Sum4/1 -> MinMax/2
  effect of inertia (Nm)/1((Nm)) -> Sum4/1
  spd command/1 -> Memory4/1, Switch1/3, Relational Operator2/1, effect of inertia (Nm)/1(req'd spd (rad/s))
  Logical Operator2/1 -> Switch2/2
  Logical Operator/1 -> Switch1/2
  no-lag Reset Integrator/1(out_1) -> Switch2/3
  just started spin-down/spin-up/1(trigger) -> no-lag Reset Integrator/2(in_2)
  Sum3/1 -> no-lag Reset Integrator/3(in_3)

== system lib_fuel_converter3/fuel converter <fc>/IC Engine Model  &  Interface/ic engine model/engine torque ==
  fc_trq_out_r : Inport
  spd command : Inport  Port=2
  engine spd : Inport  Port=3
  Block NOTES : Subsystem
      mask Display: disp('Block\nNOTES')
  Constant1 : Constant  Value=0
  Constant3 : Constant
  Logical Operator : Logic  Operator=OR
  MinMax : MinMax  Inputs=2
  MinMax1 : MinMax  Function=max  Inputs=2
  Sum : Sum  SaturateOnIntegerOverflow=on
  Sum1 : Sum  Inputs=+-  SaturateOnIntegerOverflow=on
  Switch : Switch  Threshold=eps  SaturateOnIntegerOverflow=on  InputSameDT=on
  Switch1 : Switch  Threshold=eps  SaturateOnIntegerOverflow=on  InputSameDT=on
  T_closed throttle : Subsystem
  T_max : Subsystem
  clutch not disengaged : RelationalOperator  Operator=~=  RndMeth=Nearest  InputSameDT=on
  effect of inertia (Nm) : Subsystem
  engine commanded not to decelerate : RelationalOperator  Operator=<=  RndMeth=Nearest  InputSameDT=on
  limited : RelationalOperator  Operator=~=  RndMeth=Nearest  InputSameDT=on
  map torque (Nm) : Outport
  torque to shaft (Nm) : Outport  Port=2
  tag scope: fc_trq_limited=scoped
  wires:
  Constant1/1 -> Switch1/3
  Sum1/1 -> Switch1/1
  Switch1/1 -> torque to shaft (Nm)/1
  [clutch_state] -> clutch not disengaged/1
  Constant3/1 -> clutch not disengaged/2
  engine commanded not to decelerate/1 -> Logical Operator/1
  Sum/1 -> Switch/1
  Logical Operator/1 -> Switch/2
  limited/1 -> [fc_trq_limited]
  MinMax/1 -> MinMax1/1
  T_max/1(T_max) -> MinMax/2
  T_closed throttle/1(T_closed throttle) -> Switch/3, MinMax1/2
  MinMax1/1 -> limited/2, map torque (Nm)/1, Sum1/1
  Switch/1 -> MinMax/1, limited/1
  clutch not disengaged/1 -> Switch1/2, Logical Operator/2
  engine spd/1 -> T_closed throttle/1(w_APU), T_max/1(w_APU), engine commanded not to decelerate/1, effect of inertia (Nm)/1(engine spd (rad/s))
  fc_trq_out_r/1 -> Sum/1
  effect of inertia (Nm)/1((Nm)) -> Sum/2, Sum1/2
  spd command/1 -> engine commanded not to decelerate/2

== system lib_fuel_converter3/fuel converter <fc>/IC Engine Model  &  Interface/ic engine model/enhancedToWorkspace ==
  In1 : Inport
  To Workspace : ToWorkspace  VariableName=fc_spd_out_r  SampleTime=-1
  wires:
  In1/1 -> To Workspace/1

== system lib_fuel_converter3/fuel converter <fc>/IC Engine Model  &  Interface/ic engine model/enhancedToWorkspace1 ==
  In1 : Inport
  To Workspace : ToWorkspace  VariableName=fc_spd_est  SampleTime=-1
  wires:
  In1/1 -> To Workspace/1

== system lib_fuel_converter3/fuel converter <fc>/IC Engine Model  &  Interface/ic engine model/enhancedToWorkspace3 ==
  In1 : Inport
  To Workspace : ToWorkspace  VariableName=fc_fuel  SampleTime=-1
  wires:
  In1/1 -> To Workspace/1

== system lib_fuel_converter3/fuel converter <fc>/IC Engine Model  &  Interface/ic engine model/enhancedToWorkspace4 ==
  In1 : Inport
  To Workspace : ToWorkspace  VariableName=fc_spd_out_a  SampleTime=-1
  wires:
  In1/1 -> To Workspace/1

== system lib_fuel_converter3/fuel converter <fc>/IC Engine Model  &  Interface/ic engine model/enhancedToWorkspace5 ==
  In1 : Inport
  To Workspace : ToWorkspace  VariableName=fc_trq_out_a  SampleTime=-1
  wires:
  In1/1 -> To Workspace/1

== system lib_fuel_converter3/fuel converter <fc>/IC Engine Model  &  Interface/ic engine model/enhancedToWorkspace6 ==
  In1 : Inport
  To Workspace : ToWorkspace  VariableName=fc_trq_out_r  SampleTime=-1
  wires:
  In1/1 -> To Workspace/1

== system lib_fuel_converter3/fuel converter <fc>/IC Engine Model  &  Interface/ic engine model/enhancedToWorkspace7 ==
  In1 : Inport
  To Workspace : ToWorkspace  VariableName=fc_brake_trq  SampleTime=-1
  wires:
  In1/1 -> To Workspace/1

== system lib_fuel_converter3/fuel converter <fc>/IC Engine Model  &  Interface/ic engine model/fuel use and EO emis Configurable Subsystem ==
  T (Nm) : Inport
  w (rad/s) : Inport  Port=2
  fuel use and EO emis : $bdroot/configurable subsystems/fuel use and EO emis
      settings: RTWFcnNameOpts=Auto  RTWFileNameOpts=Auto
  cumulative fuel  use (gal) : Outport
  "FC ON?, EOem, MFex, Tex, O2ex" : Outport  Port=2
  Vv,Tfc : Outport  Port=3
  wires:
  fuel use and EO emis/3 -> Vv,Tfc/1
  fuel use and EO emis/2 -> "FC ON?, EOem, MFex, Tex, O2ex"/1
  fuel use and EO emis/1 -> cumulative fuel  use (gal)/1
  w (rad/s)/1 -> fuel use and EO emis/2
  T (Nm)/1 -> fuel use and EO emis/1

== system lib_fuel_converter3/fuel converter <fc>/IC Engine Model  &  Interface/ic engine model/help ==

== system lib_fuel_converter3/fuel converter <fc> no fuel at negative torque/IC Engine Model  &  Interface/ic engine model/Block NOTES ==
  note: This block models the internal combustion engine, and includes inertia effects,
      | performance limits, accessory loads, and temperature transient effects on fuel
      | use, engine-out emissions, and catalyst efficiency.  There are 'leads' to the
      | engine controller here, which controller determines whether the engine is on.

== system lib_fuel_converter3/fuel converter <fc> no fuel at negative torque/IC Engine Model  &  Interface/ic engine model/Speed Limits ==
  Speed Requested : Inport
  Constant : Constant  Value=0
  Speed Limits : Saturate  UpperLimit=max(fc_map_spd)*fc_spd_scale  LowerLimit=vc_idle_spd*vc_idle_bool
  "if engine is not on, speed is zero" : Switch  Threshold=0.5  SaturateOnIntegerOverflow=on  InputSameDT=on
  Limited Speed Request : Outport
  wires:
  Speed Requested/1 -> Speed Limits/1
  Speed Limits/1 -> "if engine is not on, speed is zero"/1
  "if engine is not on, speed is zero"/1 -> Limited Speed Request/1
  [engine_on] -> "if engine is not on, speed is zero"/2
  Constant/1 -> "if engine is not on, speed is zero"/3
